simulink model "pole_placement_"  (R2020a)
settings: Solver=FixedStepAuto  StartTime=0.0  StopTime=100  FixedStep=1/100  RelTol=1e-3
values from neighbouring files (symbols this model uses):
  A = [ 0 1 ; 2 -1  ]    [Pole_Placement.m]    (also in Systems_Examples.m = [0 1 ; -k/m -lambda/m])
  B = [1 ; 0]    [Pole_Placement.m]    (also in Systems_Examples.m = [0 ; 1/m])
  C = [1 0]    [Pole_Placement.m]    (also in Systems_Examples.m)
  D = 0    [Pole_Placement.m]    (also in Systems_Examples.m)
  K = place(A,B,P)    [Pole_Placement.m]
  kr = 1/ dcgain(sys_cl)    [Pole_Placement.m]
settings Model: Creator=mehdi  LastModifiedBy=mehdi

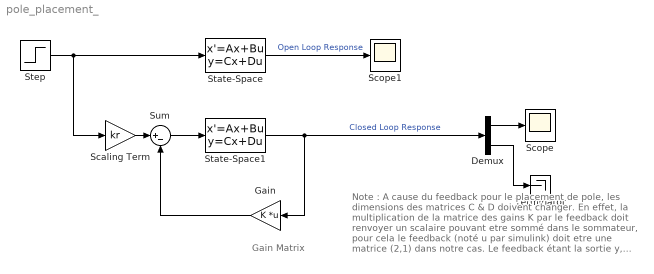
== system pole_placement_ ==
  note: Note :
      |
      | A cause du feedback pour le placement de pole, les dimensions des
      | matrices C & D doivent changer. En effet, la multiplication de la matrice
      | des gains K par le feedback doit renvoyer un scalaire pouvant etre sommé
      | dans le sommateur, pour cela le feedback (noté u par simulink) doit etre
      | une matrice (2,1) dans notre cas. Le feedback étant la sortie y, modifier les
      | dimensions de C et D nous permet d'assurer les bons calculs.
      |
      | Pour savoir quelle sortie prendre, on se refère à la matrice C originale
  note: Gain Matrix
  Demux : Demux  Outputs=2
  Gain : Gain  Gain=K  Multiplication=Matrix(K*u)
  "Scaling Term " : Gain  Gain=kr
  Scope : Scope
  Scope1 : Scope
  State-Space : StateSpace  A=A  B=B  C=C  D=D  InitialCondition=0
  State-Space1 : StateSpace  A=A  B=B  C=eye(2)  D=[0 ; 0]  InitialCondition=0
  "Step " : Step  Time=0  SampleTime=0
  Sum : Sum  Inputs=|+-
  Terminator : Terminator
  wires:
  State-Space/1 -> Scope1/1  "Open Loop Response"
  "Step "/1 -> "Scaling Term "/1, State-Space/1
  Sum/1 -> State-Space1/1
  "Scaling Term "/1 -> Sum/1
  State-Space1/1 -> Gain/1, Demux/1  "Closed Loop Response"
  Gain/1 -> Sum/2
  Demux/1 -> Scope/1
  Demux/2 -> Terminator/1
